simulink model "afe_abc_inv_psm_2mods"  (R2025b)
settings: Solver=ode1  StartTime=0.0  StopTime=simlength  FixedStep=tc  MaxStep=tc
values from neighbouring files (symbols this model uses):
  Adrso = eye(2) + Arso*ts_afe    [init_model.m]
  afe_pwm_phase_shift_mod1 = 0    [init_model.m]
  afe_pwm_phase_shift_mod2 = 0    [init_model.m]
  Aresd = eye(2) + Ares*ts_afe    [init_model.m]
  Bresd = Bres*ts_afe    [init_model.m]
  Cresd = Cres    [init_model.m]
  Crso = [1 0]    [init_model.m]
  CTRPIFF_CLIP_RELEASE = 0.001    [init_model.m]
  dead_time_AFE = 3e-6    (= 3e-06)    [init_model.m]
  dead_time_INV = 3e-6    (= 3e-06)    [init_model.m]
  deepNEGeta = 0.5    [init_model.m]
  deepNEGxi = 0    [init_model.m]
  deepPOSxi = 0.5    [init_model.m]
  emf_fb_p = 0.2    [init_model.m]
  emf_fb_p_ccaller_1 = emf_fb_p    (= 0.2)    [init_model.m]
  emf_fb_p_ccaller_2 = emf_fb_p    (= 0.2)    [init_model.m]
  emf_p = emf_fb_p*4/10    (= 0.08)    [init_model.m]
  emf_p_ccaller_1 = emf_fb_p_ccaller_1*4/10    (= 0.08)    [init_model.m]
  emf_p_ccaller_2 = emf_fb_p_ccaller_2*4/10    (= 0.08)    [init_model.m]
  fPWM_AFE = 4e3    (= 4000)    [init_model.m]
  fPWM_INV = fPWM_AFE    (= 4000)    [init_model.m]
  g0_161Hz = fcut_161Hz_flt * ts_afe * 2*pi    (= 0.126449104307)    [init_model.m]
  g0_1Hz = fcut_1Hz_flt * ts_afe * 2*pi    (= 0.000785398163397)    [init_model.m]
  g0_500Hz = fcut_500Hz_flt * ts_afe * 2*pi    (= 0.392699081699)    [init_model.m]
  g1_161Hz = 1 - g0_161Hz    (= 0.873550895693)    [init_model.m]
  g1_1Hz = 1 - g0_1Hz    (= 0.999214601837)    [init_model.m]
  g1_500Hz = 1 - g0_500Hz    (= 0.607300918301)    [init_model.m]
  i_grid_neg_eta_lim = 0.5    [init_model.m]
  i_grid_neg_eta_red_lim = 0.1    [init_model.m]
  i_grid_neg_xi_lim = 0.5    [init_model.m]
  i_grid_neg_xi_red_lim = 0.1    [init_model.m]
  i_grid_pos_eta_lim = 1    [init_model.m]
  i_grid_pos_eta_red_lim = 0.1    [init_model.m]
  id_lim = 0.35    [init_model.m]
  ieta_neg_ref_lim = 0.5    [init_model.m]
  ieta_pos_ref_lim = 1.0    (= 1)    [init_model.m]
  Igrid_phase_normalization_factor = 250e3/Vphase2/3/0.9*sqrt(2)    [init_model.m]
  inv_pwm_phase_shift_mod1 = 0    [init_model.m]
  iq_lim = 1.4    [init_model.m]
  ixi_pos_ref_lim = 1.6    [init_model.m]
  k_frt_ref = 2    [init_model.m]
  kg = Kobs(1)    [init_model.m]
  ki_afe = 45    [init_model.m]
  ki_align = 0.1    [init_model.m]
  ki_i = 18    [init_model.m]
  ki_rc_neg_grid = ki_rc_grid    (= 35)    [init_model.m]
  ki_rc_pos_grid = ki_rc_grid    (= 35)    [init_model.m]
  ki_vs = 35    [init_model.m]
  ki_w = 18    [init_model.m]
  kp_afe = 0.6    [init_model.m]
  kp_align = 0.6    [init_model.m]
  kp_i = 0.25    [init_model.m]
  kp_rc_neg_grid = kp_rc_grid    (= 0.35)    [init_model.m]
  kp_rc_pos_grid = kp_rc_grid    (= 0.35)    [init_model.m]
  kp_vs = 0.85    [init_model.m]
  kp_w = 2.5    [init_model.m]
  kw = Kobs(2)    [init_model.m]
  l1 = Kd(2)    [init_model.m]
  l2 = Kd(1)    [init_model.m]
  Ldrso = acker(Adrso',Crso',polesdrso)'    [init_model.m]
  lim_down_align = -0.2    [init_model.m]
  lim_up_align = 0.2    [init_model.m]
  mavarage_filter_frequency_base_order = 2    [init_model.m]
  motorc_m_scale = 2/3*Vdc_bez/ubez    [init_model.m]
  n1 = rms_perios/f_grid/ts_afe    [init_model.m]
  n10 = rms_perios/f_grid/ts_afe    [init_model.m]
  number_of_modules = 2    [init_model.m]
  omega_m_sim = omega_m_bez    [init_model.m]
  pll_i1 = 80    [init_model.m]
  pll_i1_ddsrt = pll_i1/2    (= 40)    [init_model.m]
  pll_p = 1    [init_model.m]
  pll_p_ddsrt = pll_p/2    (= 0.5)    [init_model.m]
  pll_p_frt = 0.2    [init_model.m]
  settle_time = 0.15    [init_model.m]
  simlength = 2    [init_model.m]
  start_time_LVRT = 2.0    (= 2)    [init_model.m]
  tc = ts_afe/200    (= 6.25e-07)    [init_model.m]
  time_aux_power_supply_fault = 1e3    (= 1000)    [init_model.m]
  time_gain_afe_module_1 = 1.0    (= 1)    [init_model.m]
  time_gain_afe_module_2 = 1.0    (= 1)    [init_model.m]
  time_gain_inv_module_1 = 1.0    (= 1)    [init_model.m]
  time_gain_inv_module_2 = 1.0    (= 1)    [init_model.m]
  time_phase_fault = 1e3    (= 1000)    [init_model.m]
  time_start_motor_control = 0.035    [init_model.m]
  transmission_delay = 125e-6*2    (= 0.00025)    [init_model.m]
  ts_afe = 1/fPWM_AFE/2    (= 0.000125)    [init_model.m]
  ts_inv = 1/fPWM_INV/2    (= 0.000125)    [init_model.m]
  Vdc_norm_ref = Vdc_ref/Vdc_nom    [init_model.m]
  Vdc_ref = 1070    [init_model.m]
  Vgrid_phase_normalization_factor = Vphase2*sqrt(2)    [init_model.m]
  w_grid = 2*pi*f_grid    [init_model.m]
undefined symbols (not defined in the file or in its folder): Amplitude_U, Amplitude_V, Amplitude_W, end_time_LVRT, ibez, La, Lb, Ld_norm, Lq_norm, Ls_norm, magnitude, omega_bez, omega_grid_emulator_nom, omega_grid_nom, omega_m_bez, Phase_shift, psi_bez, psi_m, psi_m_norm, rpm_base, rpm_bez, Rs, Rs_norm, t_ramp, tau_bez, torque_base, ubez, ugrid_factor, V_phase_normalization_factor, Vdc_bez, Vemu_ref_norm, vn_eta_pu, vn_xi_pu, vp_xi_pu
libraries: fl_lib x215, nesl_utility x107, simulink x22, cstblocks x20, threephase_inductor_lib x4, single_phase_transformer_lib x3, flexshaft_lib x1, psm x1
(part 17 of 19)

== system afe_abc_inv_psm_2mods/afe_abc_inv_psm_mod2/INV_control/inverter_control/current_ctrl/current_ctrl/dq_pi_with_vector_antiwindup mod2/dq_vector_pi_ccaller ==
  id : Inport
  id_ref : Inport  Port=2
  iq : Inport  Port=3
  iq_ref : Inport  Port=4
  udc_pu : Inport  Port=5
  Bus Selector : BusSelector  OutputSignals=ud,uq
  C Caller : CCaller  FunctionName=dqvector_pi_process_simulink  PortSpecificationStruct="%)30     .    ,!8   8    (     @         %    \"     T    !     0         %  0 \"0    $    _    07)G3F%M90  4&]R=$YA;64 4V-O<&4     26YD97@     5'EP90      4VEZ90      27-';&]B86P   X    P    !@    @    $          4    (     0    ,    !         !   P!O=70 #@   #     &    \"     0         !0    @    !     P    $         $  # &]U=  .    .     8    (    !          %    \"     $    &     0         0   ...(+7280 chars)"
  Constant : Constant  Value=ts_inv
  Constant1 : Constant  Value=kp_i
  Constant2 : Constant  Value=ki_i
  Constant3 : Constant
  Constant4 : Constant  Value=kp_i
  Constant5 : Constant  Value=ki_i
  Data Type Conversion{,1..2,4..6,9..13} (11 alike) : DataTypeConversion  OutDataTypeStr=single  SaturateOnIntegerOverflow=off  RndMeth=Floor
  Data Type Conversion3 : DataTypeConversion  OutDataTypeStr=double  SaturateOnIntegerOverflow=off  RndMeth=Floor
  Data Type Conversion7 : DataTypeConversion  OutDataTypeStr=double  SaturateOnIntegerOverflow=off  RndMeth=Floor
  Data Type Conversion8 : DataTypeConversion  OutDataTypeStr=uint8  SaturateOnIntegerOverflow=off  RndMeth=Floor
  Reset : Subsystem
  ud_ctrl_out : Outport
  uq_ctrl_out : Outport  Port=2
  wires:
  id/1 -> Data Type Conversion1/1
  id_ref/1 -> Data Type Conversion/1
  Reset/1(en) -> Data Type Conversion8/1
  iq_ref/1 -> Data Type Conversion2/1
  iq/1 -> Data Type Conversion4/1
  udc_pu/1 -> Data Type Conversion5/1
  Constant/1 -> Data Type Conversion6/1
  Constant1/1 -> Data Type Conversion9/1
  Constant2/1 -> Data Type Conversion10/1
  Constant4/1 -> Data Type Conversion13/1
  Constant5/1 -> Data Type Conversion12/1
  Constant3/1 -> Data Type Conversion11/1
  Data Type Conversion12/1 -> C Caller/11
  Data Type Conversion13/1 -> C Caller/10
  Data Type Conversion11/1 -> C Caller/12
  Data Type Conversion10/1 -> C Caller/9
  Data Type Conversion9/1 -> C Caller/8
  Data Type Conversion8/1 -> C Caller/1
  Data Type Conversion3/1 -> uq_ctrl_out/1  "uq"
  Data Type Conversion7/1 -> ud_ctrl_out/1  "ud"
  Bus Selector/1 -> Data Type Conversion7/1  "<ud>"
  Bus Selector/2 -> Data Type Conversion3/1  "<uq>"
  Data Type Conversion6/1 -> C Caller/7
  Data Type Conversion2/1 -> C Caller/4
  Data Type Conversion4/1 -> C Caller/5
  Data Type Conversion1/1 -> C Caller/3
  C Caller/1 -> Bus Selector/1  "out"
  Data Type Conversion/1 -> C Caller/2
  Data Type Conversion5/1 -> C Caller/6

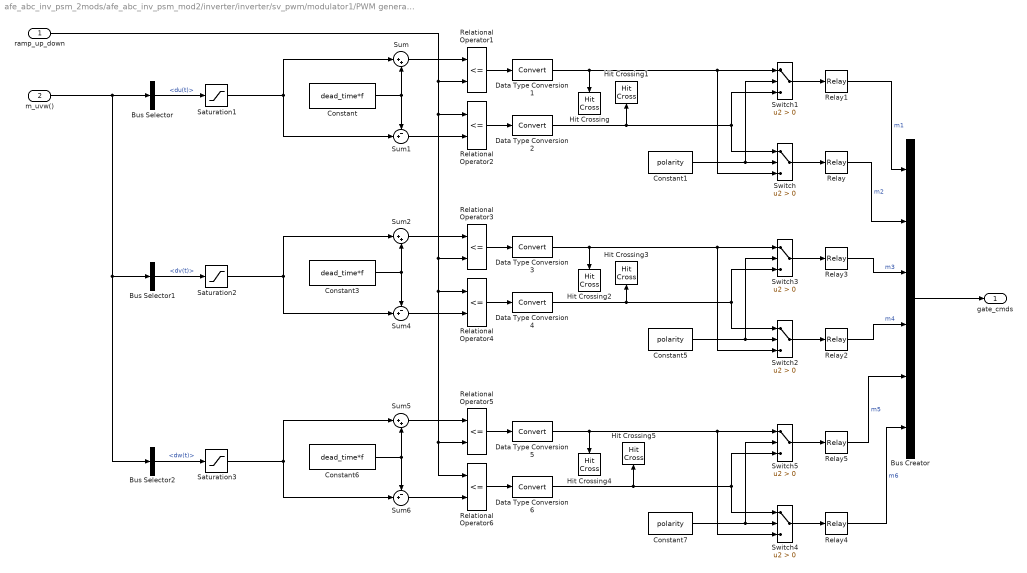
== system afe_abc_inv_psm_2mods/afe_abc_inv_psm_mod2/inverter/inverter/sv_pwm/modulator1/PWM generator/gate commands ==
  ramp_up_down : Inport
  m_uvw() : Inport  Port=2
  Bus Creator : BusCreator  Inputs=6
  Bus Selector : BusSelector  OutputSignals=du(t)
  Bus Selector1 : BusSelector  OutputSignals=dv(t)
  Bus Selector2 : BusSelector  OutputSignals=dw(t)
  Constant : Constant  Value=dead_time*f
  Constant1 : Constant  Value=polarity
  Constant3 : Constant  Value=dead_time*f
  Constant5 : Constant  Value=polarity
  Constant6 : Constant  Value=dead_time*f
  Constant7 : Constant  Value=polarity
  Data Type Conversion{1..6} (6 alike) : DataTypeConversion
  Hit Crossing{,1..5} (6 alike) : HitCross  ShowOutputPort=off
  Relational Operator{1..6} (6 alike) : RelationalOperator  Operator=<=  InputSameDT=off
  Relay{,1..5} (6 alike) : Relay  OnOutputValue=pos_cmd_gate  OffOutputValue=neg_cmd_gate
  Saturation1 : Saturate  UpperLimit=m_up  LowerLimit=m_low
  Saturation2 : Saturate  UpperLimit=m_up  LowerLimit=m_low
  Saturation3 : Saturate  UpperLimit=m_up  LowerLimit=m_low
  Sum : Sum  Inputs=|++  SaturateOnIntegerOverflow=on
  Sum1 : Sum  Inputs=-+|  SaturateOnIntegerOverflow=on
  Sum2 : Sum  Inputs=|++  SaturateOnIntegerOverflow=on
  Sum4 : Sum  Inputs=-+|  SaturateOnIntegerOverflow=on
  Sum5 : Sum  Inputs=|++  SaturateOnIntegerOverflow=on
  Sum6 : Sum  Inputs=-+|  SaturateOnIntegerOverflow=on
  Switch{,1..5} (6 alike) : Switch  Criteria=u2 > Threshold  SaturateOnIntegerOverflow=off  InputSameDT=off
  gate_cmds : Outport
  wires:
  Switch2/1 -> Relay2/1
  Relay5/1 -> Bus Creator/5  "m5"
  Constant/1 -> Sum1/1, Sum/2
  Sum6/1 -> Relational Operator6/2
  Relay1/1 -> Bus Creator/1  "m1"
  Bus Selector2/1 -> Saturation3/1  "<dw(t)>"
  Relational Operator4/1 -> Data Type Conversion4/1
  Relay/1 -> Bus Creator/2  "m2"
  Sum4/1 -> Relational Operator4/2
  Switch3/1 -> Relay3/1
  Bus Selector1/1 -> Saturation2/1  "<dv(t)>"
  Relational Operator2/1 -> Data Type Conversion2/1
  Relay3/1 -> Bus Creator/3  "m3"
  Switch1/1 -> Relay1/1
  Sum2/1 -> Relational Operator3/1
  Relational Operator3/1 -> Data Type Conversion3/1
  Saturation2/1 -> Sum2/1, Sum4/2
  Switch5/1 -> Relay5/1
  Relational Operator5/1 -> Data Type Conversion5/1
  Switch4/1 -> Relay4/1
  ramp_up_down/1 -> Relational Operator1/2, Relational Operator2/1, Relational Operator4/1, Relational Operator5/2, Relational Operator6/1, Relational Operator3/2
  Data Type Conversion4/1 -> Hit Crossing3/1, Switch3/3, Switch2/1
  Bus Selector/1 -> Saturation1/1  "<du(t)>"
  Sum5/1 -> Relational Operator5/1
  Constant7/1 -> Switch4/2, Switch5/2
  Saturation3/1 -> Sum6/2, Sum5/1
  Relay2/1 -> Bus Creator/4  "m4"
  Relational Operator6/1 -> Data Type Conversion6/1
  Sum/1 -> Relational Operator1/1
  Switch/1 -> Relay/1
  Constant5/1 -> Switch3/2, Switch2/2
  Sum1/1 -> Relational Operator2/2
  Data Type Conversion5/1 -> Hit Crossing4/1, Switch5/1, Switch4/3
  Bus Creator/1 -> gate_cmds/1
  Relational Operator1/1 -> Data Type Conversion1/1
  Data Type Conversion2/1 -> Hit Crossing1/1, Switch1/3, Switch/1
  Data Type Conversion3/1 -> Hit Crossing2/1, Switch3/1, Switch2/3
  Saturation1/1 -> Sum/1, Sum1/2
  Constant6/1 -> Sum6/1, Sum5/2
  Relay4/1 -> Bus Creator/6  "m6"
  m_uvw()/1 -> Bus Selector/1, Bus Selector1/1, Bus Selector2/1
  Constant3/1 -> Sum2/2, Sum4/1
  Data Type Conversion1/1 -> Hit Crossing/1, Switch1/1, Switch/3
  Constant1/1 -> Switch/2, Switch1/2
  Data Type Conversion6/1 -> Hit Crossing5/1, Switch5/3, Switch4/1

== system afe_abc_inv_psm_2mods/afe_abc_inv_psm_mod1/AFE_control/afe_control/grid_current_sequences_and_reactive_pwr_ctrl/current_sequence_avg/average_filter_ccaller/Moving Average Filter1/Enabled Subsystem ==
  In1 : Inport
  Enable : EnablePort
  Constant2 : Constant
  Divide : Product  Inputs=*/
  Gain1 : Gain  Gain=1/(2*pi)
  Gain9 : Gain  Gain=mavarage_filter_frequency_base_order
  Out1 : Outport
  wires:
  Gain1/1 -> Gain9/1
  Divide/1 -> Out1/1  "period"
  Gain9/1 -> Divide/2
  In1/1 -> Gain1/1  "Omega_el"
  Constant2/1 -> Divide/1

== system afe_abc_inv_psm_2mods/afe_abc_inv_psm_mod1/AFE_control/afe_control/grid_current_sequences_and_reactive_pwr_ctrl/current_sequence_avg/average_filter_ccaller/Moving Average Filter2/Enabled Subsystem ==
  In1 : Inport
  Enable : EnablePort
  Constant2 : Constant
  Divide : Product  Inputs=*/
  Gain1 : Gain  Gain=1/(2*pi)
  Gain9 : Gain  Gain=mavarage_filter_frequency_base_order
  Out1 : Outport
  wires:
  Constant2/1 -> Divide/1
  In1/1 -> Gain1/1  "Omega_el"
  Gain9/1 -> Divide/2
  Divide/1 -> Out1/1  "period"
  Gain1/1 -> Gain9/1

== system afe_abc_inv_psm_2mods/afe_abc_inv_psm_mod1/AFE_control/afe_control/grid_current_sequences_and_reactive_pwr_ctrl/current_sequence_avg/average_filter_ccaller/Moving Average Filter3/Enabled Subsystem ==
  In1 : Inport
  Enable : EnablePort
  Constant2 : Constant
  Divide : Product  Inputs=*/
  Gain1 : Gain  Gain=1/(2*pi)
  Gain9 : Gain  Gain=mavarage_filter_frequency_base_order
  Out1 : Outport
  wires:
  Gain1/1 -> Gain9/1
  Divide/1 -> Out1/1  "period"
  Gain9/1 -> Divide/2
  In1/1 -> Gain1/1  "Omega_el"
  Constant2/1 -> Divide/1

== system afe_abc_inv_psm_2mods/afe_abc_inv_psm_mod1/AFE_control/afe_control/grid_current_sequences_and_reactive_pwr_ctrl/current_sequence_avg/average_filter_ccaller/Moving Average Filter5/Enabled Subsystem ==
  In1 : Inport
  Enable : EnablePort
  Constant2 : Constant
  Divide : Product  Inputs=*/
  Gain1 : Gain  Gain=1/(2*pi)
  Gain9 : Gain  Gain=mavarage_filter_frequency_base_order
  Out1 : Outport
  wires:
  Constant2/1 -> Divide/1
  In1/1 -> Gain1/1  "Omega_el"
  Gain9/1 -> Divide/2
  Divide/1 -> Out1/1  "period"
  Gain1/1 -> Gain9/1

== system afe_abc_inv_psm_2mods/afe_abc_inv_psm_mod1/AFE_control/afe_control/grid_voltage_phase_lock_loops/DDSRF-PLL/pll_stageA/sequences/ddsrf ==
  u_grid_alpha : Inport
  u_grid_beta : Inport  Port=2
  phase_angle : Inport  Port=3
  Gain : Gain  Gain=2
  LTI System{,1..3} (4 alike) : cstblocks/LTI System  sys=ddsrf_fd  IC=[]  PadeOrder=0
  Sum : Sum  Inputs=|+-
  Sum1 : Sum  Inputs=|+-
  Sum2 : Sum  Inputs=-+|
  Sum3 : Sum  Inputs=-+|
  alphabeta2xieta_neg : MATLAB Function  TreatAsAtomicUnit=on
  alphabeta2xieta_neg1 : MATLAB Function  TreatAsAtomicUnit=on
  alphabeta2xieta_pos : MATLAB Function  TreatAsAtomicUnit=on
  alphabeta2xieta_pos1 : MATLAB Function  TreatAsAtomicUnit=on
  bounder2 : MATLAB Function  TreatAsAtomicUnit=on
  u_grid_pos_xi : Outport
  u_grid_pos_eta : Outport  Port=2
  u_grid_neg_xi : Outport  Port=3
  u_grid_neg_eta : Outport  Port=4
  wires:
  phase_angle/1 -> alphabeta2xieta_pos/3(gamma), alphabeta2xieta_neg/3(gamma), Gain/1  "phase_angle"
  u_grid_beta/1 -> alphabeta2xieta_pos/2(beta), alphabeta2xieta_neg/2(beta)  "u_grid_beta"
  u_grid_alpha/1 -> alphabeta2xieta_pos/1(alpha), alphabeta2xieta_neg/1(alpha)  "u_grid_alpha"
  alphabeta2xieta_pos/1(xi) -> Sum/1  "u_grid_pos_xi"
  Sum/1 -> LTI System/1
  alphabeta2xieta_pos/2(eta) -> Sum1/1  "u_grid_pos_eta"
  Sum1/1 -> LTI System1/1
  alphabeta2xieta_neg/1(xi) -> Sum2/2  "u_grid_neg_xi"
  Sum2/1 -> LTI System2/1
  Sum3/1 -> LTI System3/1
  alphabeta2xieta_neg/2(eta) -> Sum3/2  "u_grid_neg_eta"
  Gain/1 -> bounder2/1(u)
  LTI System/1 -> alphabeta2xieta_neg1/1(alpha), u_grid_pos_xi/1
  LTI System1/1 -> alphabeta2xieta_neg1/2(beta), u_grid_pos_eta/1
  LTI System2/1 -> u_grid_neg_xi/1, alphabeta2xieta_pos1/1(alpha)
  LTI System3/1 -> u_grid_neg_eta/1, alphabeta2xieta_pos1/2(beta)
  bounder2/1(y) -> [phase_angle_2]
  [phase_angle_2] -> alphabeta2xieta_pos1/3(gamma)
  [phase_angle_2] -> alphabeta2xieta_neg1/3(gamma)
  alphabeta2xieta_pos1/1(xi) -> Sum/2
  alphabeta2xieta_pos1/2(eta) -> Sum1/2
  alphabeta2xieta_neg1/1(xi) -> Sum2/1
  alphabeta2xieta_neg1/2(eta) -> Sum3/1

== system afe_abc_inv_psm_2mods/afe_abc_inv_psm_mod1/AFE_control/afe_control/grid_voltage_phase_lock_loops/dq_pll/pll_stageA/mormalization_and_transformation/u_500Hz_flt ==
  input : Inport
  Gain3 : Gain  Gain=g1_500Hz
  Gain6 : Gain  Gain=g0_500Hz
  Sum : Sum  Inputs=|++
  Unit Delay1 : UnitDelay  SampleTime=-1  HasFrameUpgradeWarning=on
  output : Outport  VectorParamsAs1DForOutWhenUnconnected=off
  wires:
  Sum/1 -> output/1, Unit Delay1/1
  Gain3/1 -> Sum/2
  Unit Delay1/1 -> Gain3/1
  input/1 -> Gain6/1
  Gain6/1 -> Sum/1

== system afe_abc_inv_psm_2mods/afe_abc_inv_psm_mod1/AFE_control/afe_control/grid_voltage_phase_lock_loops/dq_pll/pll_stageA/mormalization_and_transformation/u_500Hz_flt1 ==
  input : Inport
  Gain3 : Gain  Gain=g1_500Hz
  Gain6 : Gain  Gain=g0_500Hz
  Sum : Sum  Inputs=|++
  Unit Delay1 : UnitDelay  SampleTime=-1  HasFrameUpgradeWarning=on
  output : Outport  VectorParamsAs1DForOutWhenUnconnected=off
  wires:
  Gain6/1 -> Sum/1
  input/1 -> Gain6/1
  Unit Delay1/1 -> Gain3/1
  Gain3/1 -> Sum/2
  Sum/1 -> Unit Delay1/1, output/1

== system afe_abc_inv_psm_2mods/afe_abc_inv_psm_mod1/AFE_control/afe_control/grid_voltage_phase_lock_loops/dq_pll/pll_stageA/mormalization_and_transformation/u_500Hz_flt2 ==
  input : Inport
  Gain3 : Gain  Gain=g1_500Hz
  Gain6 : Gain  Gain=g0_500Hz
  Sum : Sum  Inputs=|++
  Unit Delay1 : UnitDelay  SampleTime=-1  HasFrameUpgradeWarning=on
  output : Outport  VectorParamsAs1DForOutWhenUnconnected=off
  wires:
  Sum/1 -> output/1, Unit Delay1/1
  Gain3/1 -> Sum/2
  Unit Delay1/1 -> Gain3/1
  input/1 -> Gain6/1
  Gain6/1 -> Sum/1

== system afe_abc_inv_psm_2mods/afe_abc_inv_psm_mod1/AFE_control/afe_control/grid_voltage_phase_lock_loops/dq_pll/pll_stageA/sequences/alphabeta2xieta ==
  alpha : Inport
  beta : Inport  Port=2
  gamma : Inport  Port=3
  alphabeta2xieta_neg : MATLAB Function  TreatAsAtomicUnit=on
  alphabeta2xieta_pos : MATLAB Function  TreatAsAtomicUnit=on
  xi : Outport
  eta : Outport  Port=2
  Out3 : Outport  Port=3
  Out4 : Outport  Port=4
  wires:
  alpha/1 -> alphabeta2xieta_neg/1(alpha), alphabeta2xieta_pos/1(alpha)  "u_grid_alpha"
  beta/1 -> alphabeta2xieta_neg/2(beta), alphabeta2xieta_pos/2(beta)  "u_grid_beta"
  gamma/1 -> alphabeta2xieta_neg/3(gamma), alphabeta2xieta_pos/3(gamma)  "gamma_grid"
  alphabeta2xieta_pos/1(xi) -> xi/1  "u_grid_pos_xi"
  alphabeta2xieta_pos/2(eta) -> eta/1  "u_grid_pos_eta"
  alphabeta2xieta_neg/1(xi) -> Out3/1  "u_grid_neg_xi"
  alphabeta2xieta_neg/2(eta) -> Out4/1  "u_grid_neg_eta"

== system afe_abc_inv_psm_2mods/afe_abc_inv_psm_mod1/AFE_control/afe_control/grid_voltage_sequences/voltage_sequence_avg/average_filter_ccaller/Moving Average Filter1/Enabled Subsystem ==
  In1 : Inport
  Enable : EnablePort
  Constant2 : Constant
  Divide : Product  Inputs=*/
  Gain1 : Gain  Gain=1/(2*pi)
  Gain9 : Gain  Gain=mavarage_filter_frequency_base_order
  Out1 : Outport
  wires:
  Gain1/1 -> Gain9/1
  Divide/1 -> Out1/1  "period"
  Gain9/1 -> Divide/2
  In1/1 -> Gain1/1  "Omega_el"
  Constant2/1 -> Divide/1

== system afe_abc_inv_psm_2mods/afe_abc_inv_psm_mod1/AFE_control/afe_control/grid_voltage_sequences/voltage_sequence_avg/average_filter_ccaller/Moving Average Filter2/Enabled Subsystem ==
  In1 : Inport
  Enable : EnablePort
  Constant2 : Constant
  Divide : Product  Inputs=*/
  Gain1 : Gain  Gain=1/(2*pi)
  Gain9 : Gain  Gain=mavarage_filter_frequency_base_order
  Out1 : Outport
  wires:
  Constant2/1 -> Divide/1
  In1/1 -> Gain1/1  "Omega_el"
  Gain9/1 -> Divide/2
  Divide/1 -> Out1/1  "period"
  Gain1/1 -> Gain9/1

== system afe_abc_inv_psm_2mods/afe_abc_inv_psm_mod1/AFE_control/afe_control/grid_voltage_sequences/voltage_sequence_avg/average_filter_ccaller/Moving Average Filter3/Enabled Subsystem ==
  In1 : Inport
  Enable : EnablePort
  Constant2 : Constant
  Divide : Product  Inputs=*/
  Gain1 : Gain  Gain=1/(2*pi)
  Gain9 : Gain  Gain=mavarage_filter_frequency_base_order
  Out1 : Outport
  wires:
  Gain1/1 -> Gain9/1
  Divide/1 -> Out1/1  "period"
  Gain9/1 -> Divide/2
  In1/1 -> Gain1/1  "Omega_el"
  Constant2/1 -> Divide/1

== system afe_abc_inv_psm_2mods/afe_abc_inv_psm_mod1/AFE_control/afe_control/grid_voltage_sequences/voltage_sequence_avg/average_filter_ccaller/Moving Average Filter4/Enabled Subsystem ==
  In1 : Inport
  Enable : EnablePort
  Constant2 : Constant
  Divide : Product  Inputs=*/
  Gain1 : Gain  Gain=1/(2*pi)
  Gain9 : Gain  Gain=mavarage_filter_frequency_base_order
  Out1 : Outport
  wires:
  Constant2/1 -> Divide/1
  In1/1 -> Gain1/1  "Omega_el"
  Gain9/1 -> Divide/2
  Divide/1 -> Out1/1  "period"
  Gain1/1 -> Gain9/1

== system afe_abc_inv_psm_2mods/afe_abc_inv_psm_mod1/INV_control/inverter_control/current_ctrl/bemf_observer/phase_fault/phase_fault/drop_phase_zerofor_delta_time ==
  theta_pmsm : Inport
  Product : Product
  Step : Step  Time=time_phase_fault  Before=1  After=0  SampleTime=0
  Step1 : Step  Time=time_phase_fault+3e-3  SampleTime=0
  Sum : Sum  Inputs=|++
  theta : Outport
  wires:
  theta_pmsm/1 -> Product/1
  Step1/1 -> Sum/2
  Product/1 -> theta/1
  Sum/1 -> Product/2
  Step/1 -> Sum/1

== system afe_abc_inv_psm_2mods/afe_abc_inv_psm_mod1/INV_control/inverter_control/current_ctrl/bemf_observer/phase_fault/phase_fault/hold_phase_for_delta_time ==
  theta_pmsm : Inport
  Enabled Subsystem : Subsystem  TreatAsAtomicUnit=on
  Step : Step  Time=time_phase_fault  Before=1  After=0  SampleTime=0
  Step1 : Step  Time=time_phase_fault+25e-3  SampleTime=0
  Sum : Sum  Inputs=|++
  theta : Outport
  wires:
  Step/1 -> Sum/1
  Step1/1 -> Sum/2
  theta_pmsm/1 -> Enabled Subsystem/1(theta_pmsm)
  Enabled Subsystem/1(theta) -> theta/1
  Sum/1 -> Enabled Subsystem/Enable

== system afe_abc_inv_psm_2mods/afe_abc_inv_psm_mod1/INV_control/inverter_control/current_ctrl/bemf_observer/phase_fault/phase_fault/loss_phase ==
  theta_pmsm : Inport
  Enabled Subsystem : Subsystem  TreatAsAtomicUnit=on
  Step : Step  Time=time_phase_fault  Before=1  After=0  SampleTime=0
  theta : Outport
  wires:
  Step/1 -> Enabled Subsystem/Enable
  Enabled Subsystem/1(theta) -> theta/1
  theta_pmsm/1 -> Enabled Subsystem/1(theta_pmsm)

== system afe_abc_inv_psm_2mods/afe_abc_inv_psm_mod1/INV_control/inverter_control/current_ctrl/current_ctrl/dq_pi_with_vector_antiwindup mod1/dq_vector_pi/bounder1 ==
  md : Inport
  m_1 : Inport  Port=2
  m : Inport  Port=3
  Constant : Constant
  Constant1 : Constant  Value=0
  Divide : Product
  Switch : Switch  Threshold=1  SaturateOnIntegerOverflow=off  InputSameDT=off
  Switch1 : Switch  Threshold=1  SaturateOnIntegerOverflow=off  InputSameDT=off
  md_sat : Outport  VectorParamsAs1DForOutWhenUnconnected=off
  clip : Outport  Port=2  VectorParamsAs1DForOutWhenUnconnected=off
  wires:
  md/1 -> Switch1/3, Divide/2
  m_1/1 -> Divide/1
  Divide/1 -> Switch1/1
  Switch1/1 -> md_sat/1
  Switch/1 -> clip/1
  m/1 -> Switch/2, Switch1/2
  Constant/1 -> Switch/1
  Constant1/1 -> Switch/3

== system afe_abc_inv_psm_2mods/afe_abc_inv_psm_mod1/INV_control/inverter_control/current_ctrl/current_ctrl/dq_pi_with_vector_antiwindup mod1/dq_vector_pi/bounder2 ==
  m : Inport
  m_1 : Inport  Port=2
  mq : Inport  Port=3
  Constant : Constant
  Constant1 : Constant  Value=0
  Divide : Product
  Switch : Switch  Threshold=1  SaturateOnIntegerOverflow=off  InputSameDT=off
  Switch1 : Switch  Threshold=1  SaturateOnIntegerOverflow=off  InputSameDT=off
  mq_sat : Outport  VectorParamsAs1DForOutWhenUnconnected=off
  clip : Outport  Port=2  VectorParamsAs1DForOutWhenUnconnected=off
  wires:
  Constant1/1 -> Switch/3
  Constant/1 -> Switch/1
  m/1 -> Switch1/2, Switch/2
  Switch/1 -> clip/1
  Switch1/1 -> mq_sat/1
  Divide/1 -> Switch1/1
  m_1/1 -> Divide/1
  mq/1 -> Divide/2, Switch1/3

== system afe_abc_inv_psm_2mods/afe_abc_inv_psm_mod1/INV_control/inverter_control/current_ctrl/current_ctrl/dq_pi_with_vector_antiwindup mod1/dq_vector_pi/pi_d ==
  id_tilde : Inport
  clip : Inport  Port=2
  1/Ti : Gain  Gain=kp_i  SaturateOnIntegerOverflow=on  OutDataTypeStr=Inherit: Same as input  ParamDataTypeStr=Inherit: Same as input
  Constant : Constant  Value=0
  Sum2 : Sum  Inputs=+-  SaturateOnIntegerOverflow=on
  Sum4 : Sum  SaturateOnIntegerOverflow=on
  Sum5 : Sum  SaturateOnIntegerOverflow=on
  Switch1 : Switch  Threshold=0.5  SaturateOnIntegerOverflow=off  InputSameDT=off
  Switch2 : Switch  Threshold=0.5  SaturateOnIntegerOverflow=off  InputSameDT=off
  Unit Delay1 : UnitDelay  SampleTime=-1  HasFrameUpgradeWarning=on
  Unit Delay2 : UnitDelay  SampleTime=-1  HasFrameUpgradeWarning=on
  kp1 : Gain  Gain=CTRPIFF_CLIP_RELEASE*ts_inv  SaturateOnIntegerOverflow=on  OutDataTypeStr=Inherit: Same as input  ParamDataTypeStr=Inherit: Same as input
  kp2 : Gain  Gain=ki_i*ts_inv  SaturateOnIntegerOverflow=on  OutDataTypeStr=Inherit: Same as input  ParamDataTypeStr=Inherit: Same as input
  ud_out : Outport  VectorParamsAs1DForOutWhenUnconnected=off
  wires:
  id_tilde/1 -> kp2/1, 1/Ti/1
  Sum5/1 -> ud_out/1
  Switch1/1 -> Unit Delay2/1
  Sum4/1 -> Sum5/2, Switch1/3
  kp1/1 -> Sum2/2
  Sum2/1 -> Switch1/1
  Unit Delay2/1 -> Sum4/2, kp1/1, Sum2/1
  1/Ti/1 -> Sum5/1
  Switch2/1 -> Sum4/1
  kp2/1 -> Switch2/3
  clip/1 -> Unit Delay1/1
  [clip] -> Switch2/2
  [clip] -> Switch1/2
  Constant/1 -> Switch2/1
  Unit Delay1/1 -> [clip]

== system afe_abc_inv_psm_2mods/afe_abc_inv_psm_mod1/INV_control/inverter_control/current_ctrl/current_ctrl/dq_pi_with_vector_antiwindup mod1/dq_vector_pi/pi_q ==
  iq_tilde : Inport
  clip : Inport  Port=2
  1/Ti : Gain  Gain=kp_i  SaturateOnIntegerOverflow=on  OutDataTypeStr=Inherit: Same as input  ParamDataTypeStr=Inherit: Same as input
  Constant : Constant  Value=0
  Sum2 : Sum  Inputs=+-  SaturateOnIntegerOverflow=on
  Sum4 : Sum  SaturateOnIntegerOverflow=on
  Sum5 : Sum  SaturateOnIntegerOverflow=on
  Switch1 : Switch  Threshold=0.5  SaturateOnIntegerOverflow=off  InputSameDT=off
  Switch2 : Switch  Threshold=0.5  SaturateOnIntegerOverflow=off  InputSameDT=off
  Unit Delay1 : UnitDelay  SampleTime=-1  HasFrameUpgradeWarning=on
  Unit Delay2 : UnitDelay  SampleTime=-1  HasFrameUpgradeWarning=on
  kp1 : Gain  Gain=CTRPIFF_CLIP_RELEASE*ts_inv  SaturateOnIntegerOverflow=on  OutDataTypeStr=Inherit: Same as input  ParamDataTypeStr=Inherit: Same as input
  kp2 : Gain  Gain=ki_i*ts_inv  SaturateOnIntegerOverflow=on  OutDataTypeStr=Inherit: Same as input  ParamDataTypeStr=Inherit: Same as input
  Vqs_out : Outport  VectorParamsAs1DForOutWhenUnconnected=off
  wires:
  Constant/1 -> Switch2/1
  [clip] -> Switch1/2
  [clip] -> Switch2/2
  clip/1 -> Unit Delay1/1
  kp2/1 -> Switch2/3
  Switch2/1 -> Sum4/1
  1/Ti/1 -> Sum5/1
  Unit Delay2/1 -> Sum2/1, kp1/1, Sum4/2
  Sum2/1 -> Switch1/1
  kp1/1 -> Sum2/2
  Sum4/1 -> Sum5/2, Switch1/3
  Switch1/1 -> Unit Delay2/1
  iq_tilde/1 -> 1/Ti/1, kp2/1
  Unit Delay1/1 -> [clip]
  Sum5/1 -> Vqs_out/1

== system afe_abc_inv_psm_2mods/afe_abc_inv_psm_mod1/INV_control/inverter_control/current_ctrl/current_ctrl/dq_pi_with_vector_antiwindup mod1/dq_vector_pi/switch ==
  clip 1 : Inport
  clip 2 : Inport  Port=2
  Constant4 : Constant
  Constant5 : Constant  Value=0
  Sum1 : Sum  SaturateOnIntegerOverflow=on
  Switch : Switch  Threshold=0.5  SaturateOnIntegerOverflow=off  InputSameDT=off
  clip : Outport  VectorParamsAs1DForOutWhenUnconnected=off
  wires:
  Constant5/1 -> Switch/3
  Switch/1 -> clip/1
  Constant4/1 -> Switch/1
  Sum1/1 -> Switch/2
  clip 1/1 -> Sum1/1
  clip 2/1 -> Sum1/2

== system afe_abc_inv_psm_2mods/afe_abc_inv_psm_mod1/INV_control/inverter_control/current_ctrl/current_ctrl/dq_pi_with_vector_antiwindup mod1/dq_vector_pi/vector lenght ==
  md : Inport
  mq : Inport  Port=2
  Math Function : Math  Operator=magnitude^2  SignedPower=on
  Math Function1 : Math  Operator=magnitude^2  SignedPower=on
  Math Function2 : Math  Operator=reciprocal  SignedPower=on
  Sqrt : Sqrt
  Sum5 : Sum  SaturateOnIntegerOverflow=on
  m_1 : Outport  VectorParamsAs1DForOutWhenUnconnected=off
  m : Outport  Port=2  VectorParamsAs1DForOutWhenUnconnected=off
  wires:
  Sqrt/1 -> m/1, Math Function2/1
  mq/1 -> Math Function1/1
  Math Function1/1 -> Sum5/2
  Math Function/1 -> Sum5/1
  Sum5/1 -> Sqrt/1
  Math Function2/1 -> m_1/1
  md/1 -> Math Function/1

== system afe_abc_inv_psm_2mods/afe_abc_inv_psm_mod1/INV_control/inverter_control/current_ctrl/current_ctrl/dq_pi_with_vector_antiwindup mod1/dq_vector_pi_ccaller/Reset ==
  Step : Step  Time=0.05  Before=1  After=0
  en : Outport
  wires:
  Step/1 -> en/1

== system afe_abc_inv_psm_2mods/afe_abc_inv_psm_mod2/AFE_control/afe_control/grid_current_sequences_and_reactive_pwr_ctrl/current_sequence_avg/average_filter_ccaller/Moving Average Filter1/Enabled Subsystem ==
  In1 : Inport
  Enable : EnablePort
  Constant2 : Constant
  Divide : Product  Inputs=*/
  Gain1 : Gain  Gain=1/(2*pi)
  Gain9 : Gain  Gain=mavarage_filter_frequency_base_order
  Out1 : Outport
  wires:
  Constant2/1 -> Divide/1
  In1/1 -> Gain1/1  "Omega_el"
  Gain9/1 -> Divide/2
  Divide/1 -> Out1/1  "period"
  Gain1/1 -> Gain9/1

== system afe_abc_inv_psm_2mods/afe_abc_inv_psm_mod2/AFE_control/afe_control/grid_current_sequences_and_reactive_pwr_ctrl/current_sequence_avg/average_filter_ccaller/Moving Average Filter2/Enabled Subsystem ==
  In1 : Inport
  Enable : EnablePort
  Constant2 : Constant
  Divide : Product  Inputs=*/
  Gain1 : Gain  Gain=1/(2*pi)
  Gain9 : Gain  Gain=mavarage_filter_frequency_base_order
  Out1 : Outport
  wires:
  Gain1/1 -> Gain9/1
  Divide/1 -> Out1/1  "period"
  Gain9/1 -> Divide/2
  In1/1 -> Gain1/1  "Omega_el"
  Constant2/1 -> Divide/1

== system afe_abc_inv_psm_2mods/afe_abc_inv_psm_mod2/AFE_control/afe_control/grid_current_sequences_and_reactive_pwr_ctrl/current_sequence_avg/average_filter_ccaller/Moving Average Filter3/Enabled Subsystem ==
  In1 : Inport
  Enable : EnablePort
  Constant2 : Constant
  Divide : Product  Inputs=*/
  Gain1 : Gain  Gain=1/(2*pi)
  Gain9 : Gain  Gain=mavarage_filter_frequency_base_order
  Out1 : Outport
  wires:
  Constant2/1 -> Divide/1
  In1/1 -> Gain1/1  "Omega_el"
  Gain9/1 -> Divide/2
  Divide/1 -> Out1/1  "period"
  Gain1/1 -> Gain9/1

== system afe_abc_inv_psm_2mods/afe_abc_inv_psm_mod2/AFE_control/afe_control/grid_current_sequences_and_reactive_pwr_ctrl/current_sequence_avg/average_filter_ccaller/Moving Average Filter5/Enabled Subsystem ==
  In1 : Inport
  Enable : EnablePort
  Constant2 : Constant
  Divide : Product  Inputs=*/
  Gain1 : Gain  Gain=1/(2*pi)
  Gain9 : Gain  Gain=mavarage_filter_frequency_base_order
  Out1 : Outport
  wires:
  Gain1/1 -> Gain9/1
  Divide/1 -> Out1/1  "period"
  Gain9/1 -> Divide/2
  In1/1 -> Gain1/1  "Omega_el"
  Constant2/1 -> Divide/1

== system afe_abc_inv_psm_2mods/afe_abc_inv_psm_mod2/AFE_control/afe_control/grid_voltage_phase_lock_loops/DDSRF-PLL/pll_stageA/sequences/ddsrf ==
  u_grid_alpha : Inport
  u_grid_beta : Inport  Port=2
  phase_angle : Inport  Port=3
  Gain : Gain  Gain=2
  LTI System{,1..3} (4 alike) : cstblocks/LTI System  sys=ddsrf_fd  IC=[]  PadeOrder=0
  Sum : Sum  Inputs=|+-
  Sum1 : Sum  Inputs=|+-
  Sum2 : Sum  Inputs=-+|
  Sum3 : Sum  Inputs=-+|
  alphabeta2xieta_neg : MATLAB Function  TreatAsAtomicUnit=on
  alphabeta2xieta_neg1 : MATLAB Function  TreatAsAtomicUnit=on
  alphabeta2xieta_pos : MATLAB Function  TreatAsAtomicUnit=on
  alphabeta2xieta_pos1 : MATLAB Function  TreatAsAtomicUnit=on
  bounder2 : MATLAB Function  TreatAsAtomicUnit=on
  u_grid_pos_xi : Outport
  u_grid_pos_eta : Outport  Port=2
  u_grid_neg_xi : Outport  Port=3
  u_grid_neg_eta : Outport  Port=4
  wires:
  alphabeta2xieta_neg1/2(eta) -> Sum3/1
  alphabeta2xieta_neg1/1(xi) -> Sum2/1
  alphabeta2xieta_pos1/2(eta) -> Sum1/2
  alphabeta2xieta_pos1/1(xi) -> Sum/2
  [phase_angle_2] -> alphabeta2xieta_neg1/3(gamma)
  [phase_angle_2] -> alphabeta2xieta_pos1/3(gamma)
  bounder2/1(y) -> [phase_angle_2]
  LTI System3/1 -> alphabeta2xieta_pos1/2(beta), u_grid_neg_eta/1
  LTI System2/1 -> alphabeta2xieta_pos1/1(alpha), u_grid_neg_xi/1
  LTI System1/1 -> u_grid_pos_eta/1, alphabeta2xieta_neg1/2(beta)
  LTI System/1 -> u_grid_pos_xi/1, alphabeta2xieta_neg1/1(alpha)
  Gain/1 -> bounder2/1(u)
  alphabeta2xieta_neg/2(eta) -> Sum3/2  "u_grid_neg_eta"
  Sum3/1 -> LTI System3/1
  Sum2/1 -> LTI System2/1
  alphabeta2xieta_neg/1(xi) -> Sum2/2  "u_grid_neg_xi"
  Sum1/1 -> LTI System1/1
  alphabeta2xieta_pos/2(eta) -> Sum1/1  "u_grid_pos_eta"
  Sum/1 -> LTI System/1
  alphabeta2xieta_pos/1(xi) -> Sum/1  "u_grid_pos_xi"
  u_grid_alpha/1 -> alphabeta2xieta_neg/1(alpha), alphabeta2xieta_pos/1(alpha)  "u_grid_alpha"
  u_grid_beta/1 -> alphabeta2xieta_neg/2(beta), alphabeta2xieta_pos/2(beta)  "u_grid_beta"
  phase_angle/1 -> Gain/1, alphabeta2xieta_neg/3(gamma), alphabeta2xieta_pos/3(gamma)  "phase_angle"

== system afe_abc_inv_psm_2mods/afe_abc_inv_psm_mod2/AFE_control/afe_control/grid_voltage_phase_lock_loops/dq_pll/pll_stageA/mormalization_and_transformation/u_500Hz_flt ==
  input : Inport
  Gain3 : Gain  Gain=g1_500Hz
  Gain6 : Gain  Gain=g0_500Hz
  Sum : Sum  Inputs=|++
  Unit Delay1 : UnitDelay  SampleTime=-1  HasFrameUpgradeWarning=on
  output : Outport  VectorParamsAs1DForOutWhenUnconnected=off
  wires:
  Gain6/1 -> Sum/1
  input/1 -> Gain6/1
  Unit Delay1/1 -> Gain3/1
  Gain3/1 -> Sum/2
  Sum/1 -> Unit Delay1/1, output/1

== system afe_abc_inv_psm_2mods/afe_abc_inv_psm_mod2/AFE_control/afe_control/grid_voltage_phase_lock_loops/dq_pll/pll_stageA/mormalization_and_transformation/u_500Hz_flt1 ==
  input : Inport
  Gain3 : Gain  Gain=g1_500Hz
  Gain6 : Gain  Gain=g0_500Hz
  Sum : Sum  Inputs=|++
  Unit Delay1 : UnitDelay  SampleTime=-1  HasFrameUpgradeWarning=on
  output : Outport  VectorParamsAs1DForOutWhenUnconnected=off
  wires:
  Sum/1 -> output/1, Unit Delay1/1
  Gain3/1 -> Sum/2
  Unit Delay1/1 -> Gain3/1
  input/1 -> Gain6/1
  Gain6/1 -> Sum/1

== system afe_abc_inv_psm_2mods/afe_abc_inv_psm_mod2/AFE_control/afe_control/grid_voltage_phase_lock_loops/dq_pll/pll_stageA/mormalization_and_transformation/u_500Hz_flt2 ==
  input : Inport
  Gain3 : Gain  Gain=g1_500Hz
  Gain6 : Gain  Gain=g0_500Hz
  Sum : Sum  Inputs=|++
  Unit Delay1 : UnitDelay  SampleTime=-1  HasFrameUpgradeWarning=on
  output : Outport  VectorParamsAs1DForOutWhenUnconnected=off
  wires:
  Gain6/1 -> Sum/1
  input/1 -> Gain6/1
  Unit Delay1/1 -> Gain3/1
  Gain3/1 -> Sum/2
  Sum/1 -> Unit Delay1/1, output/1

== system afe_abc_inv_psm_2mods/afe_abc_inv_psm_mod2/AFE_control/afe_control/grid_voltage_phase_lock_loops/dq_pll/pll_stageA/sequences/alphabeta2xieta ==
  alpha : Inport
  beta : Inport  Port=2
  gamma : Inport  Port=3
  alphabeta2xieta_neg : MATLAB Function  TreatAsAtomicUnit=on
  alphabeta2xieta_pos : MATLAB Function  TreatAsAtomicUnit=on
  xi : Outport
  eta : Outport  Port=2
  Out3 : Outport  Port=3
  Out4 : Outport  Port=4
  wires:
  alphabeta2xieta_neg/2(eta) -> Out4/1  "u_grid_neg_eta"
  alphabeta2xieta_neg/1(xi) -> Out3/1  "u_grid_neg_xi"
  alphabeta2xieta_pos/2(eta) -> eta/1  "u_grid_pos_eta"
  alphabeta2xieta_pos/1(xi) -> xi/1  "u_grid_pos_xi"
  gamma/1 -> alphabeta2xieta_pos/3(gamma), alphabeta2xieta_neg/3(gamma)  "gamma_grid"
  beta/1 -> alphabeta2xieta_pos/2(beta), alphabeta2xieta_neg/2(beta)  "u_grid_beta"
  alpha/1 -> alphabeta2xieta_pos/1(alpha), alphabeta2xieta_neg/1(alpha)  "u_grid_alpha"

== system afe_abc_inv_psm_2mods/afe_abc_inv_psm_mod2/AFE_control/afe_control/grid_voltage_sequences/voltage_sequence_avg/average_filter_ccaller/Moving Average Filter1/Enabled Subsystem ==
  In1 : Inport
  Enable : EnablePort
  Constant2 : Constant
  Divide : Product  Inputs=*/
  Gain1 : Gain  Gain=1/(2*pi)
  Gain9 : Gain  Gain=mavarage_filter_frequency_base_order
  Out1 : Outport
  wires:
  Constant2/1 -> Divide/1
  In1/1 -> Gain1/1  "Omega_el"
  Gain9/1 -> Divide/2
  Divide/1 -> Out1/1  "period"
  Gain1/1 -> Gain9/1

== system afe_abc_inv_psm_2mods/afe_abc_inv_psm_mod2/AFE_control/afe_control/grid_voltage_sequences/voltage_sequence_avg/average_filter_ccaller/Moving Average Filter2/Enabled Subsystem ==
  In1 : Inport
  Enable : EnablePort
  Constant2 : Constant
  Divide : Product  Inputs=*/
  Gain1 : Gain  Gain=1/(2*pi)
  Gain9 : Gain  Gain=mavarage_filter_frequency_base_order
  Out1 : Outport
  wires:
  Gain1/1 -> Gain9/1
  Divide/1 -> Out1/1  "period"
  Gain9/1 -> Divide/2
  In1/1 -> Gain1/1  "Omega_el"
  Constant2/1 -> Divide/1

== system afe_abc_inv_psm_2mods/afe_abc_inv_psm_mod2/AFE_control/afe_control/grid_voltage_sequences/voltage_sequence_avg/average_filter_ccaller/Moving Average Filter3/Enabled Subsystem ==
  In1 : Inport
  Enable : EnablePort
  Constant2 : Constant
  Divide : Product  Inputs=*/
  Gain1 : Gain  Gain=1/(2*pi)
  Gain9 : Gain  Gain=mavarage_filter_frequency_base_order
  Out1 : Outport
  wires:
  Constant2/1 -> Divide/1
  In1/1 -> Gain1/1  "Omega_el"
  Gain9/1 -> Divide/2
  Divide/1 -> Out1/1  "period"
  Gain1/1 -> Gain9/1

== system afe_abc_inv_psm_2mods/afe_abc_inv_psm_mod2/AFE_control/afe_control/grid_voltage_sequences/voltage_sequence_avg/average_filter_ccaller/Moving Average Filter4/Enabled Subsystem ==
  In1 : Inport
  Enable : EnablePort
  Constant2 : Constant
  Divide : Product  Inputs=*/
  Gain1 : Gain  Gain=1/(2*pi)
  Gain9 : Gain  Gain=mavarage_filter_frequency_base_order
  Out1 : Outport
  wires:
  Gain1/1 -> Gain9/1
  Divide/1 -> Out1/1  "period"
  Gain9/1 -> Divide/2
  In1/1 -> Gain1/1  "Omega_el"
  Constant2/1 -> Divide/1

== system afe_abc_inv_psm_2mods/afe_abc_inv_psm_mod2/INV_control/inverter_control/current_ctrl/bemf_observer/phase_fault/phase_fault/drop_phase_zerofor_delta_time ==
  theta_pmsm : Inport
  Product : Product
  Step : Step  Time=time_phase_fault  Before=1  After=0  SampleTime=0
  Step1 : Step  Time=time_phase_fault+3e-3  SampleTime=0
  Sum : Sum  Inputs=|++
  theta : Outport
  wires:
  Step/1 -> Sum/1
  Sum/1 -> Product/2
  Product/1 -> theta/1
  Step1/1 -> Sum/2
  theta_pmsm/1 -> Product/1

== system afe_abc_inv_psm_2mods/afe_abc_inv_psm_mod2/INV_control/inverter_control/current_ctrl/bemf_observer/phase_fault/phase_fault/hold_phase_for_delta_time ==
  theta_pmsm : Inport
  Enabled Subsystem : Subsystem  TreatAsAtomicUnit=on
  Step : Step  Time=time_phase_fault  Before=1  After=0  SampleTime=0
  Step1 : Step  Time=time_phase_fault+25e-3  SampleTime=0
  Sum : Sum  Inputs=|++
  theta : Outport
  wires:
  Sum/1 -> Enabled Subsystem/Enable
  Enabled Subsystem/1(theta) -> theta/1
  theta_pmsm/1 -> Enabled Subsystem/1(theta_pmsm)
  Step1/1 -> Sum/2
  Step/1 -> Sum/1

== system afe_abc_inv_psm_2mods/afe_abc_inv_psm_mod2/INV_control/inverter_control/current_ctrl/bemf_observer/phase_fault/phase_fault/loss_phase ==
  theta_pmsm : Inport
  Enabled Subsystem : Subsystem  TreatAsAtomicUnit=on
  Step : Step  Time=time_phase_fault  Before=1  After=0  SampleTime=0
  theta : Outport
  wires:
  theta_pmsm/1 -> Enabled Subsystem/1(theta_pmsm)
  Enabled Subsystem/1(theta) -> theta/1
  Step/1 -> Enabled Subsystem/Enable

== system afe_abc_inv_psm_2mods/afe_abc_inv_psm_mod2/INV_control/inverter_control/current_ctrl/current_ctrl/dq_pi_with_vector_antiwindup mod2/dq_vector_pi/bounder1 ==
  md : Inport
  m_1 : Inport  Port=2
  m : Inport  Port=3
  Constant : Constant
  Constant1 : Constant  Value=0
  Divide : Product
  Switch : Switch  Threshold=1  SaturateOnIntegerOverflow=off  InputSameDT=off
  Switch1 : Switch  Threshold=1  SaturateOnIntegerOverflow=off  InputSameDT=off
  md_sat : Outport  VectorParamsAs1DForOutWhenUnconnected=off
  clip : Outport  Port=2  VectorParamsAs1DForOutWhenUnconnected=off
  wires:
  Constant1/1 -> Switch/3
  Constant/1 -> Switch/1
  m/1 -> Switch1/2, Switch/2
  Switch/1 -> clip/1
  Switch1/1 -> md_sat/1
  Divide/1 -> Switch1/1
  m_1/1 -> Divide/1
  md/1 -> Divide/2, Switch1/3

== system afe_abc_inv_psm_2mods/afe_abc_inv_psm_mod2/INV_control/inverter_control/current_ctrl/current_ctrl/dq_pi_with_vector_antiwindup mod2/dq_vector_pi/bounder2 ==
  m : Inport
  m_1 : Inport  Port=2
  mq : Inport  Port=3
  Constant : Constant
  Constant1 : Constant  Value=0
  Divide : Product
  Switch : Switch  Threshold=1  SaturateOnIntegerOverflow=off  InputSameDT=off
  Switch1 : Switch  Threshold=1  SaturateOnIntegerOverflow=off  InputSameDT=off
  mq_sat : Outport  VectorParamsAs1DForOutWhenUnconnected=off
  clip : Outport  Port=2  VectorParamsAs1DForOutWhenUnconnected=off
  wires:
  mq/1 -> Switch1/3, Divide/2
  m_1/1 -> Divide/1
  Divide/1 -> Switch1/1
  Switch1/1 -> mq_sat/1
  Switch/1 -> clip/1
  m/1 -> Switch/2, Switch1/2
  Constant/1 -> Switch/1
  Constant1/1 -> Switch/3

== system afe_abc_inv_psm_2mods/afe_abc_inv_psm_mod2/INV_control/inverter_control/current_ctrl/current_ctrl/dq_pi_with_vector_antiwindup mod2/dq_vector_pi/pi_d ==
  id_tilde : Inport
  clip : Inport  Port=2
  1/Ti : Gain  Gain=kp_i  SaturateOnIntegerOverflow=on  OutDataTypeStr=Inherit: Same as input  ParamDataTypeStr=Inherit: Same as input
  Constant : Constant  Value=0
  Sum2 : Sum  Inputs=+-  SaturateOnIntegerOverflow=on
  Sum4 : Sum  SaturateOnIntegerOverflow=on
  Sum5 : Sum  SaturateOnIntegerOverflow=on
  Switch1 : Switch  Threshold=0.5  SaturateOnIntegerOverflow=off  InputSameDT=off
  Switch2 : Switch  Threshold=0.5  SaturateOnIntegerOverflow=off  InputSameDT=off
  Unit Delay1 : UnitDelay  SampleTime=-1  HasFrameUpgradeWarning=on
  Unit Delay2 : UnitDelay  SampleTime=-1  HasFrameUpgradeWarning=on
  kp1 : Gain  Gain=CTRPIFF_CLIP_RELEASE*ts_inv  SaturateOnIntegerOverflow=on  OutDataTypeStr=Inherit: Same as input  ParamDataTypeStr=Inherit: Same as input
  kp2 : Gain  Gain=ki_i*ts_inv  SaturateOnIntegerOverflow=on  OutDataTypeStr=Inherit: Same as input  ParamDataTypeStr=Inherit: Same as input
  ud_out : Outport  VectorParamsAs1DForOutWhenUnconnected=off
  wires:
  Unit Delay1/1 -> [clip]
  Constant/1 -> Switch2/1
  [clip] -> Switch1/2
  [clip] -> Switch2/2
  clip/1 -> Unit Delay1/1
  kp2/1 -> Switch2/3
  Switch2/1 -> Sum4/1
  1/Ti/1 -> Sum5/1
  Unit Delay2/1 -> Sum2/1, kp1/1, Sum4/2
  Sum2/1 -> Switch1/1
  kp1/1 -> Sum2/2
  Sum4/1 -> Switch1/3, Sum5/2
  Switch1/1 -> Unit Delay2/1
  Sum5/1 -> ud_out/1
  id_tilde/1 -> 1/Ti/1, kp2/1
